simulink model "observador"  (R2018a)
settings: Solver=VariableStepAuto  StartTime=0.0  StopTime=10.0  RelTol=1e-3
values from neighbouring files (symbols this model uses):
  b_eq = b_m + b_l/r^2    (= 1.5e-05)    [proyecto_global_integrador.m]
  J_eq = J_m + J_l/r^2    (= 5.65099476805e-06)    [proyecto_global_integrador.m]
  Ke_theta = 9597.74    [proyecto_global_integrador.m]
  Ke_w = 30699997.7    [proyecto_global_integrador.m]
settings Model: Creator=gabrielq  LastModifiedBy=gabrielq

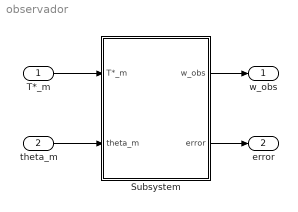
== system observador ==
  "T*_m " : Inport
  "theta_m " : Inport  Port=2
  Subsystem : Subsystem
  "w_obs " : Outport
  "error " : Outport  Port=2
  wires:
  "T*_m "/1 -> Subsystem/1("T*_m ")
  "theta_m "/1 -> Subsystem/2("theta_m ")
  Subsystem/1("w_obs ") -> "w_obs "/1
  Subsystem/2("error ") -> "error "/1

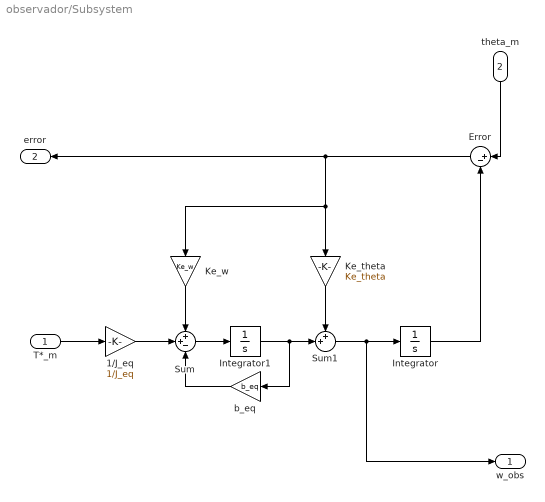
== system observador/Subsystem ==
  "T*_m " : Inport
  "theta_m " : Inport  Port=2
  1/J_eq : Gain  Gain=1/J_eq
  "Error " : Sum  Inputs=|+-
  Integrator : Integrator
  Integrator1 : Integrator
  Ke_theta : Gain  Gain=Ke_theta
  "Ke_w " : Gain  Gain=Ke_w
  Sum : Sum  Inputs=++-
  Sum1 : Sum  Inputs=++|
  b_eq : Gain  Gain=b_eq
  "w_obs " : Outport
  "error " : Outport  Port=2
  wires:
  "T*_m "/1 -> 1/J_eq/1
  Sum/1 -> Integrator1/1
  Integrator/1 -> "Error "/2
  "theta_m "/1 -> "Error "/1
  Sum1/1 -> "w_obs "/1, Integrator/1
  Integrator1/1 -> b_eq/1, Sum1/2
  "Error "/1 -> "error "/1, "Ke_w "/1, Ke_theta/1
  Ke_theta/1 -> Sum1/1
  "Ke_w "/1 -> Sum/1
  1/J_eq/1 -> Sum/2
  b_eq/1 -> Sum/3
